simulink model "butter_fil"  (R2020b)
settings: Solver=VariableStepAuto  StartTime=0.0  StopTime=0.01  RelTol=1e-3
values from neighbouring files (symbols this model uses):
  fs = 100e6    (= 100000000)    [read_ila_data.m]    (also in signal_generation.m = 10000000; signal_line.mat = 10000000)
libraries: simulink x1, fillib x1
settings Model: Creator=pablo  LastModifiedBy=pablo

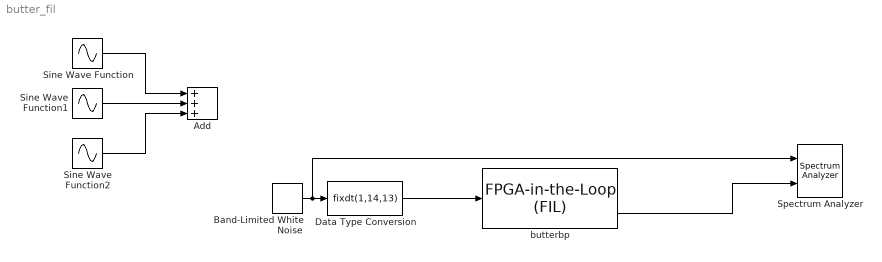
== system butter_fil ==
  Add : Sum  Inputs=+++
  Band-Limited White Noise : simulink/Sources/Band-Limited White Noise  Cov=[0.000001]  Ts=1/fs  seed=[23341]
  Data Type Conversion : DataTypeConversion  OutDataTypeStr=fixdt(1,14,13)
  Sine Wave Function : Sin  Amplitude=0.3  Frequency=2*pi*900e3  SampleTime=1/fs
  Sine Wave Function1 : Sin  Amplitude=0.3  Frequency=2*pi*1000e3  SampleTime=1/fs
  Sine Wave Function2 : Sin  Amplitude=0.3  Frequency=2*pi*1100e3  SampleTime=1/fs
  Spectrum Analyzer : SpectrumAnalyzer  NumInputPorts=2
  butterbp : fillib/FPGA-in-the-Loop (FIL)  ForceInterfaceUpdate=0.44968
      settings: SourceProductBaseCode=ES,HD
  wires:
  Data Type Conversion/1 -> butterbp/1
  butterbp/2 -> Spectrum Analyzer/2
  Sine Wave Function1/1 -> Add/2
  Sine Wave Function/1 -> Add/1
  Sine Wave Function2/1 -> Add/3
  Band-Limited White Noise/1 -> Spectrum Analyzer/1, Data Type Conversion/1
